simulink model "part1_1_m3"  (R2019b)
settings: Solver=VariableStepAuto  StartTime=-1  StopTime=1  RelTol=1e-3
settings Model: Creator=SEFA  LastModifiedBy=SEFA

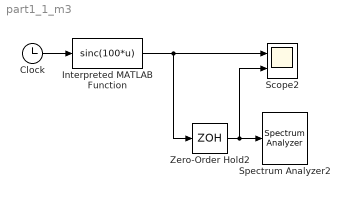
== system part1_1_m3 ==
  Clock : Clock
  Interpreted MATLAB Function : MATLABFcn  MATLABFcn=sinc(100*u)
  Scope2 : Scope  NumInputPorts=2
  Spectrum Analyzer2 : SpectrumAnalyzer
  Zero-Order Hold2 : ZeroOrderHold  SampleTime=1/2000
  wires:
  Zero-Order Hold2/1 -> Scope2/2, Spectrum Analyzer2/1
  Clock/1 -> Interpreted MATLAB Function/1
  Interpreted MATLAB Function/1 -> Zero-Order Hold2/1, Scope2/1
